simulink model "inverseTest"  (R2018b)
settings: Solver=ode4  StartTime=0.0  StopTime=300  FixedStep=0.02  RelTol=1e-3
undefined symbols (not defined in the file): SS_discrete, SS_full, SS_inverse
settings Model: Creator=user  LastModifiedBy=user

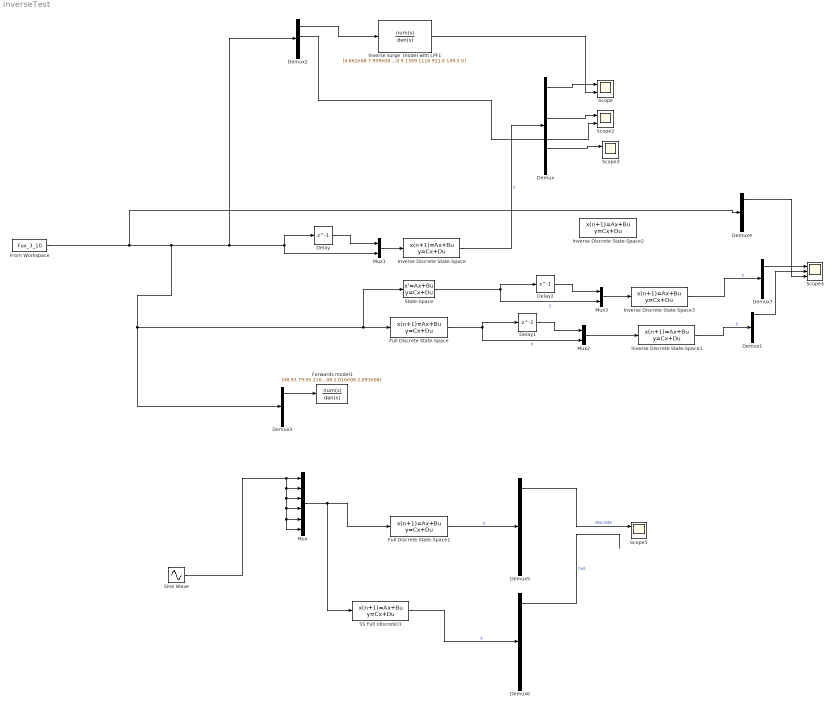
== system inverseTest ==
  Delay : Delay  DelayLength=1  InitialCondition=0
  Delay1 : Delay  DelayLength=1  InitialCondition=0
  Delay2 : Delay  DelayLength=1  InitialCondition=0
  Demux{,1..7} (8 alike) : Demux  Outputs=6
  Forwards model1 : TransferFcn  Numerator=[48.93 79.95 216.2 144.3 149.5 0]  Denominator=[9.724e07 1.592e08 5.128e08 4.252e08 6.336e08 2.016e08 2.093e08]
  From Workspace : FromWorkspace  VariableName=Fex_3_10
  Full Discrete State-Space : DiscreteStateSpace  A=SS_discrete.A  B=SS_discrete.B  C=SS_discrete.C  D=SS_discrete.D  SampleTime=0.02
  Full Discrete State-Space1 : DiscreteStateSpace  A=SS_discrete.A  B=SS_discrete.B  C=SS_discrete.C  D=SS_discrete.D  SampleTime=-1
  Inverse Discrete State-Space{,1..3} (4 alike) : DiscreteStateSpace  A=SS_inverse.A  B=SS_inverse.B  C=SS_inverse.C  D=SS_inverse.D  SampleTime=-1
  Inverse surge  model with LPF1 : TransferFcn  Numerator=[4.862e08 7.959e08 2.564e09 2.126e09 3.168e09 1.008e09 1.046e09 0]  Denominator=[48.93 334.4 680.9 1349 1116 921.6 149.5 0]
  Mux : Mux  Inputs=6
  Mux1 : Mux  Inputs=2
  Mux2 : Mux  Inputs=2
  Mux3 : Mux  Inputs=2
  SS Full (discrete)1 : DiscreteStateSpace  A=SS_full.A  B=SS_full.B  C=SS_full.C  D=SS_full.D  SampleTime=-1
  Scope{,2..3,5} (4 alike) : Scope  NumInputPorts=2
  Scope4 : Scope  NumInputPorts=3
  Sine Wave : Sin  Amplitude=3e5  Frequency=2*pi  SampleTime=0
  State-Space : StateSpace  A=SS_full.A  B=SS_full.B  C=SS_full.C  D=SS_full.D  InitialCondition=0
  wires:
  Demux/1 -> Scope/1
  From Workspace/1 -> Demux4/1, State-Space/1, Full Discrete State-Space/1, Demux3/1, Demux2/1, Mux1/2, Delay/1
  Mux1/1 -> Inverse Discrete State-Space/1
  Inverse Discrete State-Space/1 -> Demux/1  "y"
  Delay/1 -> Mux1/1
  Demux/3 -> Scope2/1
  Demux1/1 -> Scope4/2
  Full Discrete State-Space/1 -> Mux2/2, Delay1/1  "y"
  Demux/5 -> Scope3/1
  Inverse surge  model with LPF1/1 -> Scope/2
  Demux2/1 -> Inverse surge  model with LPF1/1
  Demux3/1 -> Forwards model1/1
  Demux2/3 -> Scope2/2
  Full Discrete State-Space1/1 -> Demux5/1  "y"
  SS Full (discrete)1/1 -> Demux6/1  "y"
  Sine Wave/1 -> Mux/6, Mux/5, Mux/4, Mux/3, Mux/2, Mux/1
  Mux/1 -> SS Full (discrete)1/1, Full Discrete State-Space1/1
  Demux5/1 -> Scope5/1  "Discrete"
  Demux6/1 -> ?  "Full"
  Demux7/1 -> Scope4/1
  Inverse Discrete State-Space1/1 -> Demux1/1  "y"
  Delay1/1 -> Mux2/1
  Mux2/1 -> Inverse Discrete State-Space1/1
  Inverse Discrete State-Space3/1 -> Demux7/1  "y"
  State-Space/1 -> Mux3/2, Delay2/1  "y"
  Delay2/1 -> Mux3/1
  Mux3/1 -> Inverse Discrete State-Space3/1
  Demux4/1 -> Scope4/3
